simulink model "ADCS"  (R2018a)
settings: Solver=VariableStepAuto  StartTime=0.0  StopTime=600  RelTol=1e-3
settings Model: Creator=hridu  LastModifiedBy=Hridu

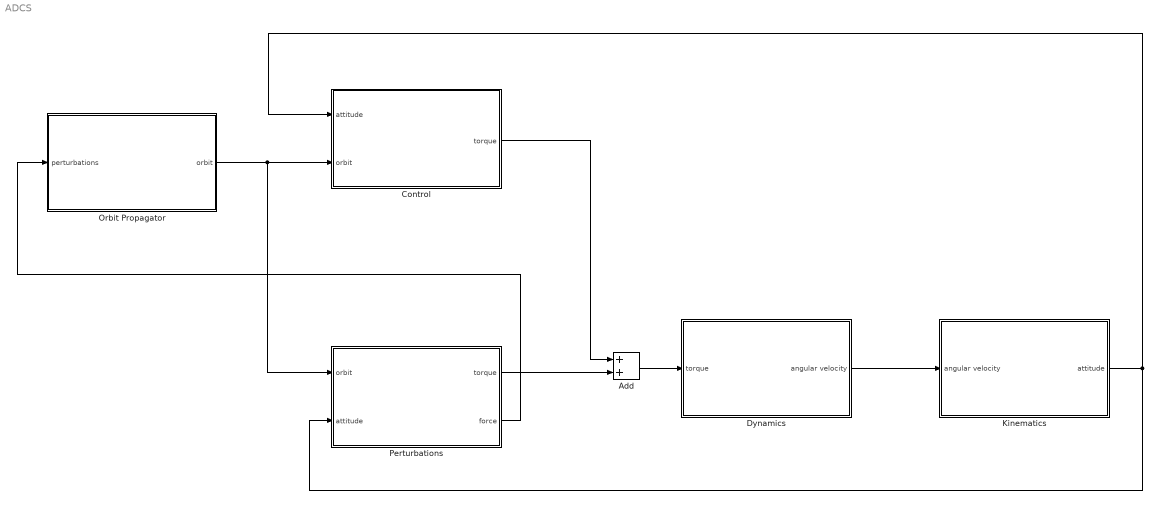
== system ADCS ==
  Add : Sum
  Control : Subsystem
  Dynamics : Subsystem
  Kinematics : Subsystem
  Orbit Propagator : Subsystem
  Perturbations : Subsystem
  wires:
  Dynamics/1(angular velocity) -> Kinematics/1(angular velocity)
  Orbit Propagator/1(orbit) -> Control/2(orbit), Perturbations/1(orbit)
  Kinematics/1(attitude) -> Perturbations/2(attitude), Control/1(attitude)
  Control/1(torque) -> Add/1
  Perturbations/1(torque) -> Add/2
  Add/1 -> Dynamics/1(torque)
  Perturbations/2(force) -> Orbit Propagator/1(perturbations)

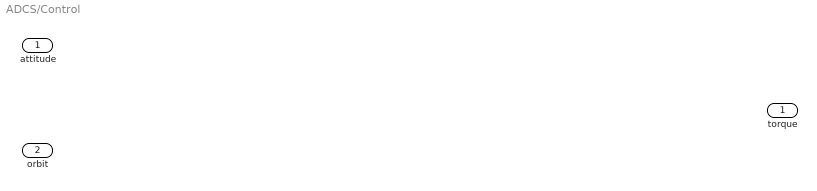
== system ADCS/Control ==
  attitude : Inport
  orbit : Inport  Port=2
  torque : Outport

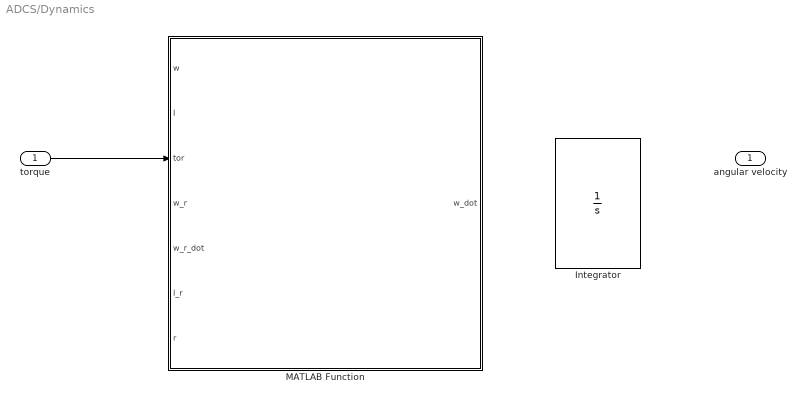
== system ADCS/Dynamics ==
  torque : Inport
  Integrator : Integrator
  MATLAB Function : MATLAB Function  TreatAsAtomicUnit=on
  angular velocity : Outport
  wires:
  torque/1 -> MATLAB Function/3(tor)

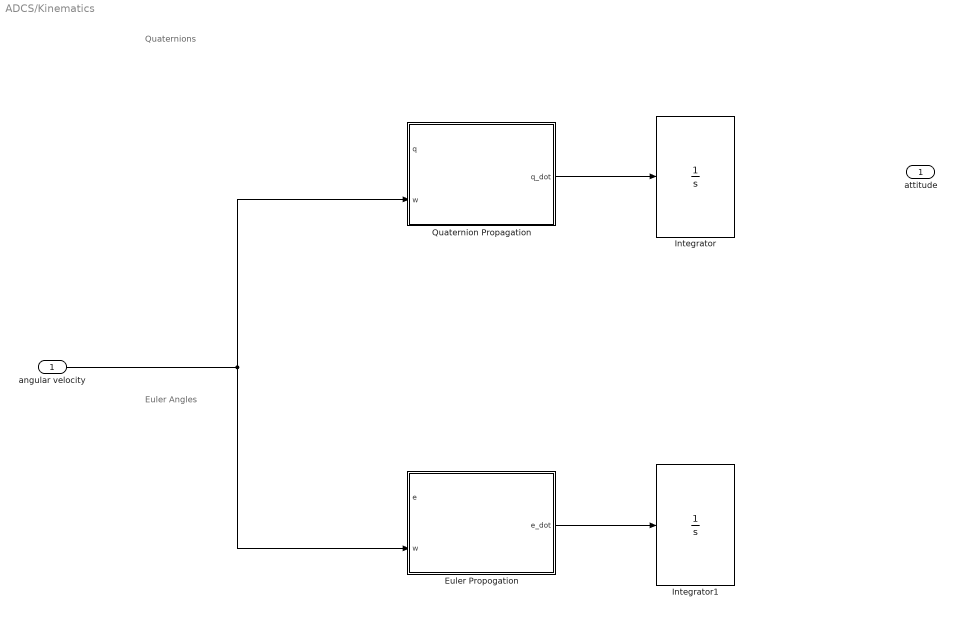
== system ADCS/Kinematics ==
  note: Euler Angles
  note: Quaternions
  angular velocity : Inport
  Euler Propogation : MATLAB Function  TreatAsAtomicUnit=on
  Integrator : Integrator
  Integrator1 : Integrator
  Quaternion Propagation : MATLAB Function  TreatAsAtomicUnit=on
  attitude : Outport
  wires:
  angular velocity/1 -> Euler Propogation/2(w), Quaternion Propagation/2(w)
  Euler Propogation/1(e_dot) -> Integrator1/1
  Quaternion Propagation/1(q_dot) -> Integrator/1

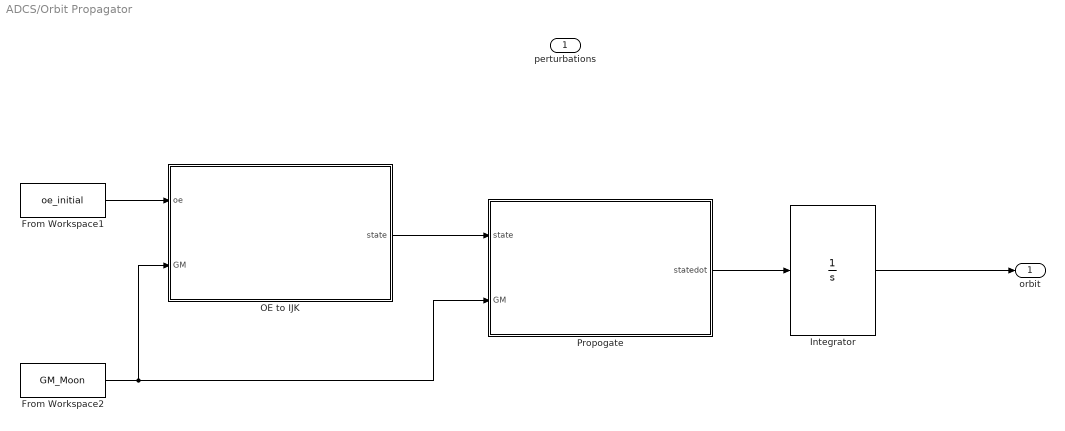
== system ADCS/Orbit Propagator ==
  perturbations : Inport
  From Workspace1 : FromWorkspace  VariableName=oe_initial  SampleTime=0
  From Workspace2 : FromWorkspace  VariableName=GM_Moon  SampleTime=0
  Integrator : Integrator
  OE to IJK : MATLAB Function  TreatAsAtomicUnit=on
  Propogate : MATLAB Function  TreatAsAtomicUnit=on
  orbit : Outport
  wires:
  From Workspace1/1 -> OE to IJK/1(oe)
  OE to IJK/1(state) -> Propogate/1(state)
  From Workspace2/1 -> Propogate/2(GM), OE to IJK/2(GM)
  Propogate/1(statedot) -> Integrator/1
  Integrator/1 -> orbit/1

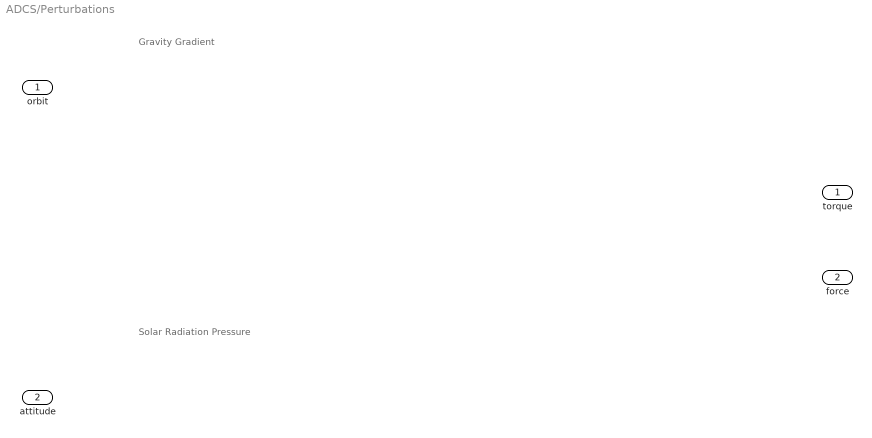
== system ADCS/Perturbations ==
  note: Gravity Gradient
  note: Solar Radiation Pressure
  orbit : Inport
  attitude : Inport  Port=2
  torque : Outport
  force : Outport  Port=2

== matlab function ADCS/Kinematics/Euler Propogation ==
  data: e input; e_dot output; w input
function e_dot   = calc_e_dot( e, w )
%INPUT: euler angles, angular velocity
%OUTPUT: rate of change of euler angles
%propagate actual dynamics
    tan_the = tan(e(2));
    if(abs(tan_the) > 300) %make sure tan(theta) is well defined
        tan_the = 300*sign(tan_the);
        disp('tan x')
    end
    cos_the = cos(e(2));
    if(abs(cos_the) < 10^-4) %make sure cos(theta) is well defined
        cos_the = 10^-4*sign(cos_the);
        disp('cos x')
    end
    A = [1, tan_the*sin(e(1)), tan_the*cos(e(1));
         0, cos(e(1)),              -1*sin(e(1));
         0, sin(e(1))/cos_the,  cos(e(1))/cos_the];
    e_dot = A*w;
end

== matlab function ADCS/Dynamics/MATLAB Function ==
  data: w input; w_dot output; I input; tor input; w_r input; w_r_dot input; I_r input; r input
function w_dot = calc_w_dot(w, I, tor, w_r, w_r_dot, I_r, r)
    %w_dot without rotor
    w_dot(1, 1) = (tor(1) - (I(3,3)-I(2,2))*w(2)*w(3))/I(1,1);
    w_dot(2, 1) = (tor(2) - (I(1,1)-I(3,3))*w(3)*w(1))/I(2,2);
    w_dot(3, 1) = (tor(3) - (I(2,2)-I(1,1))*w(1)*w(2))/I(3,3);
    
    %w_dot with rotor, assume rotor speed is constant or w_r_dot is known
    wrx = I_r*w_r_dot*r(1) + I_r*w_r*(w(2)*r(3) - w(3)*r(2));
    wry = I_r*w_r_dot*r(2) + I_r*w_r*(w(3)*r(1) - w(1)*r(3));
    wrz = I_r*w_r_dot*r(3) + I_r*w_r*(w(1)*r(2) - w(2)*r(1));
    w_dot(1, 1) = (tor(1) - (I(3,3)-I(2,2))*w(2)*w(3) - wrx) /I(1,1);
    w_dot(2, 1) = (tor(2) - (I(1,1)-I(3,3))*w(3)*w(1) - wry) /I(2,2);
    w_dot(3, 1) = (tor(3) - (I(2,2)-I(1,1))*w(1)*w(2) - wrz) /I(3,3);
end

== matlab function ADCS/Orbit Propagator/Propogate ==
  data: statedot output; state input; GM input
function statedot = accelPointMass(state, GM)
statedot = zeros(6,1);
statedot(1:3) = state(4:6);
statedot(4:6) = -GM*state(1:3)./norm(state(1:3))^3;
end

== matlab function ADCS/Kinematics/Quaternion Propagation ==
  data: q input; q_dot output; w input
function q_dot = calc_q_dot(q, w) 
%v1, not working so well
%     eta=q(1);
%     e1 =q(2);
%     e2 =q(3);
%     e3 =q(4);
%     e=[e1;e2;e3];   %euler axis
%     eta_dot=-1/2*e'*w;
%     e_dot= 1/2*(eta*eye(3)+Skew(e))*w; %euler angle
%     q_dot=[eta_dot; e_dot];

%v2, try DAmico's notes
wx = w(1); wy = w(2); wz = w(3);
OMEGA = [   0,    wz, -1*wy, wx;
        -1*wz,     0,    wx, wy;
           wy, -1*wx,     0, wz;
        -1*wx, -1*wy, -1*wz,  0];
q_dot = 0.5*OMEGA*q;
end

== matlab function ADCS/Orbit Propagator/OE to IJK ==
  data: state output; oe input; GM input
function state = kep2rv(oe, GM)
    % Function converts orbital elements to [r,v]. All angles should be in ...
    %       [rad]. oe = [a,e,i,Omega,omega,nu]
    
    %Parsing Inputs:
    a = oe(1);
    e = oe(2);
    inc = oe(3);
    raan = oe(4);
    arg = oe(5);
    nu = oe(6);
    
    % Parameters
    T = 2*pi*sqrt((a^3)/(GM)); %[s]
    n = 2*pi/T; %[rad/s]
    
    % Rotation matrix calculation
    rot = Rz(-raan)*Rx(-inc)*Rz(-arg);
    
    E = 2*atan(sqrt((1-e)/(1+e))*tan(nu/2));
    
    % Perifocal vectors calculation
    rpqw = [a*(cos(E)-e); a*sin(E)*sqrt(1-(e^2)); 0];
    vpqw = (a*n/(1-e*cos(E)))*[-sin(E) cos(E)*sqrt(1-e^2) 0]';
    
    % ECI vectors calculation
    rijk = rot*rpqw;
    vijk = rot*vpqw;
    state = [rijk; vijk];
end

function R = Rz(th)
    %Calculates the rotation matrix for rotation about Z-axis
    R = [cos(th) sin(th) 0;...
        -sin(th) cos(th) 0;...
        0 0 1];
end

function R = Rx(th)
    %Calculates the rotation matrix for rotation about X-axis
    R = [1 0 0;...
        0 cos(th) sin(th);...
        0 -sin(th) cos(th)];
end
